simulink model "plant2016_cybership"  (R2015b)
settings: Solver=VariableStepAuto  SolverMode=SingleTasking  StartTime=0.0  StopTime=300  FixedStep=.01  RelTol=1e-3  AbsTol=1e-6
StartFcn:
  | %plot_Contr_index('open')
libraries: simulink x7
(part 1 of 2)
CloseFcn:
  | ;slview('closediagram',bdroot);
settings Model: ExtModeTrigMode=oneshot  ExtModeArmWhenConnect=off  Creator=mjun  LastModifiedBy=TordFO
settings DataIOCC: LimitDataPoints=off  SaveFormat=Array  SignalLoggingSaveFormat=ModelDataLogs  SaveOutput=off  SaveTime=off
settings OptimizationCC: BlockReduction=off  BooleanDataType=off
settings DebuggingCC: SaveWithParameterizedLinksMsg=none  UnderspecifiedInitializationDetection=Classic  MergeDetectMultiDrivingBlocksExec=none  SignalResolutionControl=TryResolveAllWithWarning  MultiTaskDSMMsg=warning  MultiTaskCondExecSysMsg=none
settings HardwareCC: ProdBitPerPointer=32  ProdLargestAtomicFloat=None  ProdIntDivRoundTo=Undefined  ProdEndianess=Unspecified  ProdWordSize=32  ProdHWDeviceType=32-bit Generic  TargetUnknown=on
settings RTWCC: TemplateMakefile=grt_unix.tmf
settings GRTTargetCC: GeneratePreprocessorConditionals=Disable all  CombineOutputUpdateFcns=off  GRTInterface=on
settings ConfigComp: CovModelRefEnable=Off  CovSFcnEnable=off

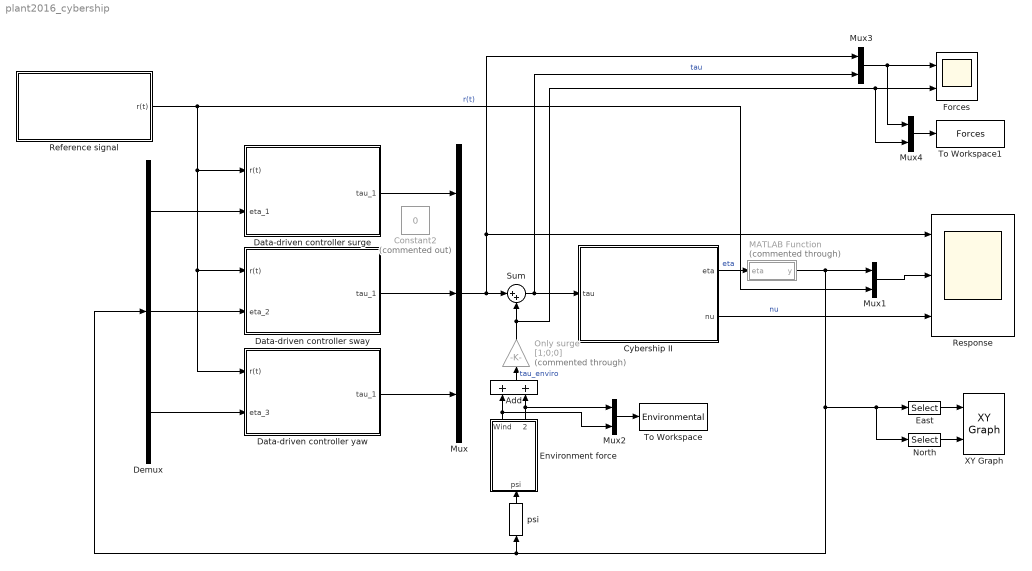
== system plant2016_cybership ==
  Add : Sum
  Constant2 : Constant  Commented=on  Value=0
  Cybership II : Subsystem
  Data-driven controller surge : Subsystem
  Data-driven controller sway : Subsystem
  Data-driven controller yaw : Subsystem
  Demux : Demux  Outputs=3
  East : Selector  InputPortWidth=3  IndexOptions=Index vector (dialog)  Indices=[2]  OutputSizes=1
  Environment force : Subsystem
  Forces : Scope  NumInputPorts=2
  MATLAB Function : MATLAB Function  Commented=through  TreatAsAtomicUnit=on
  Mux : Mux  Inputs=3
  Mux{1..4} (4 alike) : Mux  Inputs=2
  North : Selector  InputPortWidth=3  IndexOptions=Index vector (dialog)  Indices=[1]  OutputSizes=1
  Only surge : Gain  Commented=through  Gain=[1;0;0]
  Reference signal : Subsystem
  Response : Scope  NumInputPorts=3
  Sum : Sum  Inputs=|++
  To Workspace : ToWorkspace  VariableName=Environmental  SaveFormat=Timeseries  SampleTime=-1
  To Workspace1 : ToWorkspace  VariableName=Forces  SaveFormat=Timeseries  SampleTime=-1
  XY Graph : simulink/Sinks/XY Graph  xmin=-1  xmax=1  ymin=-1  ymax=1  st=-1
  psi : Selector  InputPortWidth=3  IndexOptions=Index vector (dialog)  Indices=3  OutputSizes=1
  wires:
  Reference signal/1(r(t)) -> Mux1/2, Data-driven controller sway/1(r(t)), Data-driven controller yaw/1(r(t)), Data-driven controller surge/1(r(t))  "r(t)"
  Mux/1 -> Sum/1, Mux3/1, Response/1
  Cybership II/2(nu) -> Response/3  "nu"
  Demux/3 -> Data-driven controller yaw/2(eta_3)
  Demux/1 -> Data-driven controller surge/2(eta_1)
  Mux1/1 -> Response/2
  Sum/1 -> Mux3/2, Cybership II/1(tau)  "tau"
  Environment force/1(Wind) -> Mux2/2, Add/1
  Environment force/2(Waves) -> Add/2, Mux2/1
  North/1 -> XY Graph/2
  East/1 -> XY Graph/1
  Mux2/1 -> To Workspace/1
  Mux3/1 -> Mux4/1, Forces/1
  Mux4/1 -> To Workspace1/1
  Add/1 -> Only surge/1  "tau_enviro"
  Demux/2 -> Data-driven controller sway/2(eta_2)
  Cybership II/1(eta) -> MATLAB Function/1(eta)  "eta"
  Only surge/1 -> Mux4/2, Forces/2, Sum/2
  Data-driven controller surge/1(tau_1) -> Mux/1
  MATLAB Function/1(y) -> Mux1/1, psi/1, Demux/1, North/1, East/1
  psi/1 -> Environment force/1(psi)
  Data-driven controller yaw/1(tau_1) -> Mux/3
  Data-driven controller sway/1(tau_1) -> Mux/2

== system plant2016_cybership/Cybership II ==
  tau : Inport
  Integrator : Integrator  InitialCondition=[0 0 0]'
  Integrator1 : Integrator  InitialCondition=[0.1;0;0]
  MATLAB Function : MATLAB Function  TreatAsAtomicUnit=on
  Memory : Memory
  Path calculator : MATLAB Function  TreatAsAtomicUnit=on
  Selector : Selector  InputPortWidth=3  IndexOptions=Index vector (dialog)  Indices=3  OutputSizes=1
  To Workspace1 : ToWorkspace  VariableName=nu_dot  SaveFormat=Timeseries  SampleTime=-1
  eta_dot : MATLAB Function  TreatAsAtomicUnit=on
  eta : Outport
  nu : Outport  Port=2
  wires:
  tau/1 -> Path calculator/1(tau)
  eta_dot/1(eta_dot) -> MATLAB Function/1(eta)  "eta_dot"
  Path calculator/1(nu_dot) -> To Workspace1/1, Integrator/1  "nu_dot"
  Integrator1/1 -> Selector/1, eta/1  "eta"
  Integrator/1 -> nu/1, Path calculator/2(nu), eta_dot/2(nu)  "nu"
  Selector/1 -> Memory/1  "psi"
  Memory/1 -> eta_dot/1(psi)  "psi"
  MATLAB Function/1(y) -> Integrator1/1

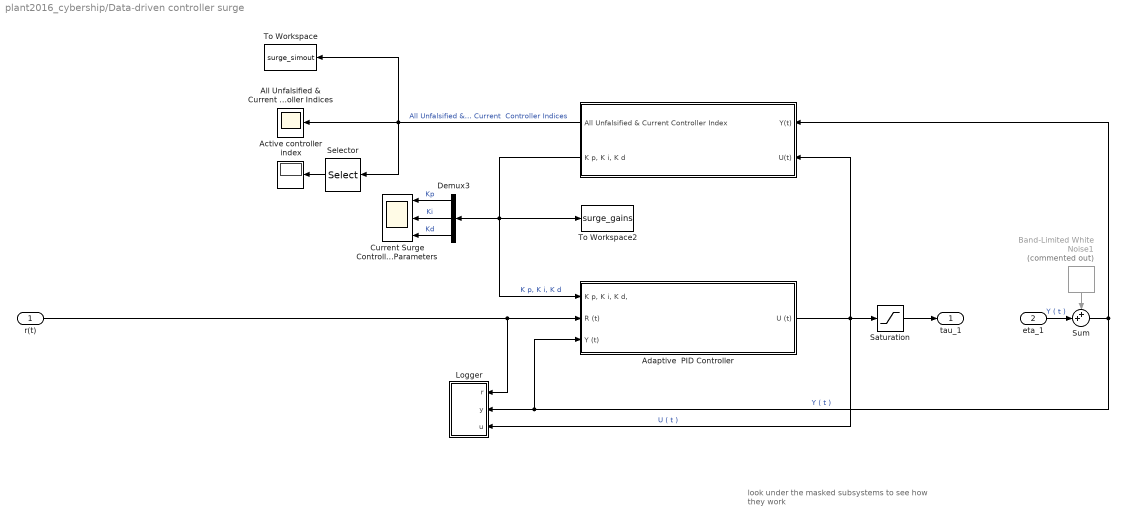
== system plant2016_cybership/Data-driven controller surge ==
  note: look under the masked subsystems
      |  to see how they work
  r(t) : Inport
  eta_1 : Inport  Port=2
  " " : Subsystem  Priority=1  mask(Unfalsification Algorithm){w1_n=1.*[1 20], w1_d=2*[1 3], w2_n=0.01, w2_d=1.2*[1 3 3 1], C_p=[10 100], C_i=[1  20], C_d=[15 20], rho=0.1}
      mask prompts: w1_n "Numerater of filter W1"; w1_d "Denominater of filter W1"; w2_n "Numerater of filter W2"; w2_d "Denominater of filter W2"; C_p "Set of proportional gains, (horizontal vector)"; C_i "Set of integral gains, (horizontal vector)"; C_d "Set of derivative gains, (horizontal vector)"; rho "Set cost-limit"
      mask help:
      | Look under the mask see how "Unfalsification Algorithm" works.
      |
      | Initially, from U & Y, the S-function "fic_ref" generates online the ficticious reference signal for all Candidate Controllers. The S-function "cost_func" then calculates the cost/ performance index for each candidate controllers. Then, based on these Performance Indices, the unfalsification algorithm selects the optimal controller for every instant and outputs the controller parameter ( in our case which is the value of Kp, Ki, Kd).
      |
      | The initilization command of this block calls a m-file "initilization". This m-file sets the port size of the mux & demux blocks inside the subsystem to the number of initial candidate controller whenever the user changes the set of initial condidate controller from the parameter entry block of this subsystem.
      |
      | Original filter-parameters:
      | w1_num =   [1 20]
      | w1_dem = 2*[1 3]
      | w2_num = 0.01
      | w2_den = 1.2*[1 3 3 1]
      mask init:
      | surge_initialization
      mask Help:
      | Look under the mask see how "Unfalsification Algorithm" works.
      | Initially, from U & Y, the S-function "fic_ref" generates online the ficticious reference signal for all Candidate Controllers.
      | The S-function "cost_func" then calculates the cost/ performance index for each candidate controllers.
      | Then, based on these Performance Indices, the S-Function "Supervisor.m" selects the optimal controller for every instant and outputs the controller parameter ( in our case which is the value of Kp, Ki, Kd).
      | The initilization command of this block calls a m-file "initilization". This m-file sets the port size of the mux & demux blocks inside the subsystem to the number of initial candidate controller whenever the user changes the set of initial condidate controller from the parameter entry block of this subsystem.
      mask Display: disp('Unfalsification Algorithm')
  Active controller index : Display
  Adaptive  PID Controller : Subsystem  mask(Adaptive PID Controller){Epsilon=.01, Delta=.010}
      mask prompts: Delta "Sampling time"
      mask init:
      | global epsilon delta
      | epsilon=Epsilon; delta = Delta;
      mask Help: This is an Adaptive PID Controller subsystem. The PID controller parameter (Kp, Ki, Kd) is determined at each instant by the Unfalsification algorithm. Look under the mask to see how this block works. The initilization commands of this block declares "epsilon" & "delta" as global variables. "epsilon" is the time-constant for approximate derivative and "delta" is the sampling time for all s-functions. Other S-functions under the Unfalsification Subsystem access these 2 variables by declaring them as global in their respective m-files.
      mask Display: disp('Adaptive PID Controller')
  All Unfalsified & Current Controller Indices : Scope
      settings: Tag=cont_plot
  Band-Limited White Noise1 : simulink/Sources/Band-Limited White Noise  Commented=on  Cov=[0.00001]  Ts=0.01  seed=[23341]
  Current Surge Controller Parameters : Scope  NumInputPorts=3
  Demux3 : Demux  Outputs=3
  Logger : Subsystem
  Saturation : Saturate  UpperLimit=10  LowerLimit=-10
  Selector : Selector  IndexOptions=Index vector (dialog)  Indices=[1]  OutputSizes=1
  Sum : Sum  Inputs=++|
  To Workspace : ToWorkspace  VariableName=surge_simout  SaveFormat=Timeseries  SampleTime=-1
  To Workspace2 : ToWorkspace  VariableName=surge_gains  SaveFormat=Timeseries  SampleTime=-1
  tau_1 : Outport
  wires:
  " "/1(All Unfalsified & Current Controller Index) -> To Workspace/1, All Unfalsified & Current Controller Indices/1, Selector/1  "All Unfalsified & Current  Controller Indices"
  Adaptive  PID Controller/1(U (t)) -> " "/2(U(t)), Logger/3(u), Saturation/1  "U ( t )"
  " "/2("K p, K i, K d") -> Adaptive  PID Controller/1("K p, K i, K d,"), To Workspace2/1, Demux3/1  "K p, K i, K d"
  Sum/1 -> " "/1(Y(t)), Logger/2(y), Adaptive  PID Controller/3(Y (t))  "Y ( t )"
  Demux3/1 -> Current Surge Controller Parameters/1  "Kp"
  r(t)/1 -> Adaptive  PID Controller/2(R (t)), Logger/1(r)
  eta_1/1 -> Sum/2  "Y ( t )"
  Demux3/2 -> Current Surge Controller Parameters/2  "Ki"
  Band-Limited White Noise1/1 -> Sum/1
  Demux3/3 -> Current Surge Controller Parameters/3  "Kd"
  Selector/1 -> Active controller index/1
  Saturation/1 -> tau_1/1

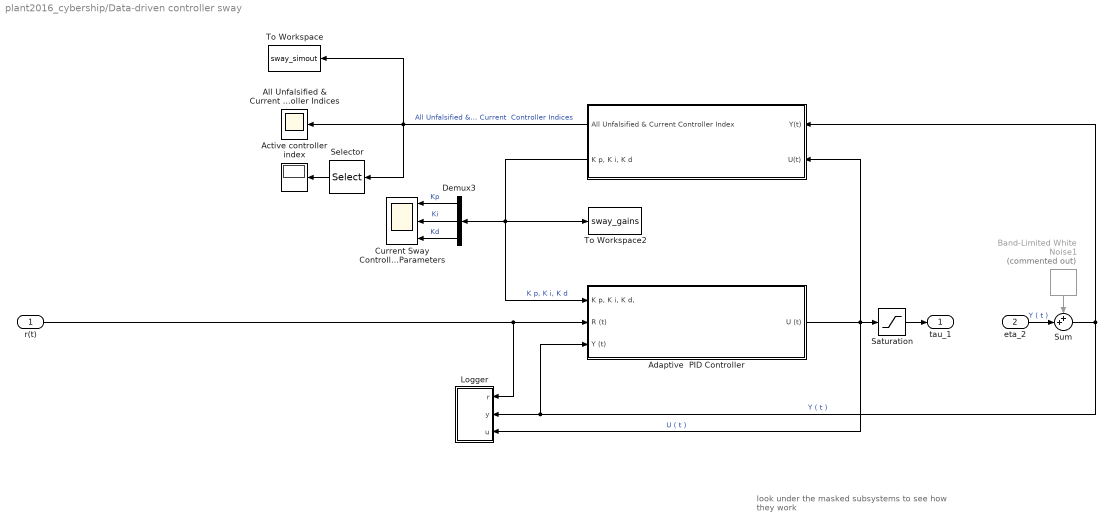
== system plant2016_cybership/Data-driven controller sway ==
  note: look under the masked subsystems
      |  to see how they work
  r(t) : Inport
  eta_2 : Inport  Port=2
  " " : Subsystem  Priority=1  mask(Unfalsification Algorithm){w1_n=1.*[1 20], w1_d=2*[1 3], w2_n=0.01, w2_d=1.2*[1 3 3 1], C_p=[10 150], C_i=[5 10], C_d=[5 10], rho=0.5}
      mask prompts: w1_n "Numerater of filter W1"; w1_d "Denominater of filter W1"; w2_n "Numerater of filter W2"; w2_d "Denominater of filter W2"; C_p "Set of proportional gains, (horizontal vector)"; C_i "Set of integral gains, (horizontal vector)"; C_d "Set of derivative gains, (horizontal vector)"; rho "Set cost-limit"
      mask help:
      | Look under the mask see how "Unfalsification Algorithm" works.
      |
      | Initially, from U & Y, the S-function "fic_ref" generates online the ficticious reference signal for all Candidate Controllers. The S-function "cost_func" then calculates the cost/ performance index for each candidate controllers. Then, based on these Performance Indices, the unfalsification algorithm selects the optimal controller for every instant and outputs the controller parameter ( in our case which is the value of Kp, Ki, Kd).
      |
      | The initilization command of this block calls a m-file "initilization". This m-file sets the port size of the mux & demux blocks inside the subsystem to the number of initial candidate controller whenever the user changes the set of initial condidate controller from the parameter entry block of this subsystem.
      |
      | Original filter-parameters:
      | w1_num =   [1 20]
      | w1_dem = 2*[1 3]
      | w2_num = 0.01
      | w2_den = 1.2*[1 3 3 1]
      mask init:
      | sway_initialization
      mask Help:
      | Look under the mask see how "Unfalsification Algorithm" works.
      | Initially, from U & Y, the S-function "fic_ref" generates online the ficticious reference signal for all Candidate Controllers.
      | The S-function "cost_func" then calculates the cost/ performance index for each candidate controllers.
      | Then, based on these Performance Indices, the S-Function "Supervisor.m" selects the optimal controller for every instant and outputs the controller parameter ( in our case which is the value of Kp, Ki, Kd).
      | The initilization command of this block calls a m-file "initilization". This m-file sets the port size of the mux & demux blocks inside the subsystem to the number of initial candidate controller whenever the user changes the set of initial condidate controller from the parameter entry block of this subsystem.
      mask Display: disp('Unfalsification Algorithm')
  Active controller index : Display
  Adaptive  PID Controller : Subsystem  mask(Adaptive PID Controller){Epsilon=.01, Delta=.01}
      mask prompts: Delta "Sampling time"
      mask init:
      | global epsilon delta
      | epsilon=Epsilon; delta = Delta;
      mask Help: This is an Adaptive PID Controller subsystem. The PID controller parameter (Kp, Ki, Kd) is determined at each instant by the Unfalsification algorithm. Look under the mask to see how this block works. The initilization commands of this block declares "epsilon" & "delta" as global variables. "epsilon" is the time-constant for approximate derivative and "delta" is the sampling time for all s-functions. Other S-functions under the Unfalsification Subsystem access these 2 variables by declaring them as global in their respective m-files.
      mask Display: disp('Adaptive PID Controller')
  All Unfalsified & Current Controller Indices : Scope
      settings: Tag=cont_plot
  Band-Limited White Noise1 : simulink/Sources/Band-Limited White Noise  Commented=on  Cov=[0.00001]  Ts=0.01  seed=[23341]
  Current Sway Controller Parameters : Scope  NumInputPorts=3
  Demux3 : Demux  Outputs=3
  Logger : Subsystem
  Saturation : Saturate  UpperLimit=10  LowerLimit=-10
  Selector : Selector  IndexOptions=Index vector (dialog)  Indices=[1]  OutputSizes=1
  Sum : Sum  Inputs=++|
  To Workspace : ToWorkspace  VariableName=sway_simout  SaveFormat=Timeseries  SampleTime=-1
  To Workspace2 : ToWorkspace  VariableName=sway_gains  SaveFormat=Timeseries  SampleTime=-1
  tau_1 : Outport
  wires:
  Selector/1 -> Active controller index/1
  Demux3/3 -> Current Sway Controller Parameters/3  "Kd"
  Band-Limited White Noise1/1 -> Sum/1
  Demux3/2 -> Current Sway Controller Parameters/2  "Ki"
  eta_2/1 -> Sum/2  "Y ( t )"
  r(t)/1 -> Logger/1(r), Adaptive  PID Controller/2(R (t))
  Demux3/1 -> Current Sway Controller Parameters/1  "Kp"
  Sum/1 -> " "/1(Y(t)), Adaptive  PID Controller/3(Y (t)), Logger/2(y)  "Y ( t )"
  " "/2("K p, K i, K d") -> Demux3/1, To Workspace2/1, Adaptive  PID Controller/1("K p, K i, K d,")  "K p, K i, K d"
  Adaptive  PID Controller/1(U (t)) -> " "/2(U(t)), Saturation/1, Logger/3(u)  "U ( t )"
  " "/1(All Unfalsified & Current Controller Index) -> Selector/1, All Unfalsified & Current Controller Indices/1, To Workspace/1  "All Unfalsified & Current  Controller Indices"
  Saturation/1 -> tau_1/1

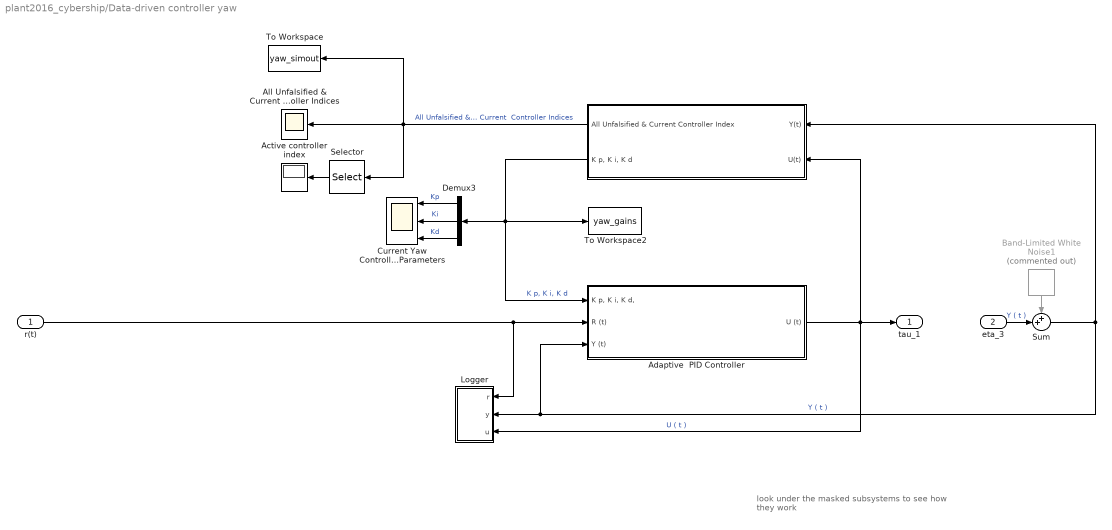
== system plant2016_cybership/Data-driven controller yaw ==
  note: look under the masked subsystems
      |  to see how they work
  r(t) : Inport
  eta_3 : Inport  Port=2
  " " : Subsystem  Priority=1  mask(Unfalsification Algorithm){w1_n=1.*[1 20], w1_d=2*[1 3], w2_n=0.01, w2_d=1.2*[1 3 3 1], C_p=[5 10 20 ], C_i=[1 8], C_d=[5 10], rho=0.2}
      mask prompts: w1_n "Numerater of filter W1"; w1_d "Denominater of filter W1"; w2_n "Numerater of filter W2"; w2_d "Denominater of filter W2"; C_p "Set of proportional gains, (horizontal vector)"; C_i "Set of integral gains, (horizontal vector)"; C_d "Set of derivative gains, (horizontal vector)"; rho "Set cost-limit"
      mask help:
      | Look under the mask see how "Unfalsification Algorithm" works.
      |
      | Initially, from U & Y, the S-function "fic_ref" generates online the ficticious reference signal for all Candidate Controllers. The S-function "cost_func" then calculates the cost/ performance index for each candidate controllers. Then, based on these Performance Indices, the unfalsification algorithm selects the optimal controller for every instant and outputs the controller parameter ( in our case which is the value of Kp, Ki, Kd).
      |
      | The initilization command of this block calls a m-file "initilization". This m-file sets the port size of the mux & demux blocks inside the subsystem to the number of initial candidate controller whenever the user changes the set of initial condidate controller from the parameter entry block of this subsystem.
      |
      | Original filter-parameters:
      | w1_num =   [1 20]
      | w1_dem = 2*[1 3]
      | w2_num = 0.01
      | w2_den = 1.2*[1 3 3 1]
      mask init:
      | yaw_initialization
      mask Help:
      | Look under the mask see how "Unfalsification Algorithm" works.
      | Initially, from U & Y, the S-function "fic_ref" generates online the ficticious reference signal for all Candidate Controllers.
      | The S-function "cost_func" then calculates the cost/ performance index for each candidate controllers.
      | Then, based on these Performance Indices, the S-Function "Supervisor.m" selects the optimal controller for every instant and outputs the controller parameter ( in our case which is the value of Kp, Ki, Kd).
      | The initilization command of this block calls a m-file "initilization". This m-file sets the port size of the mux & demux blocks inside the subsystem to the number of initial candidate controller whenever the user changes the set of initial condidate controller from the parameter entry block of this subsystem.
      mask Display: disp('Unfalsification Algorithm')
  Active controller index : Display
  Adaptive  PID Controller : Subsystem  mask(Adaptive PID Controller){Epsilon=.01, Delta=.01}
      mask prompts: Delta "Sampling time"
      mask init:
      | global epsilon delta
      | epsilon=Epsilon; delta = Delta;
      mask Help: This is an Adaptive PID Controller subsystem. The PID controller parameter (Kp, Ki, Kd) is determined at each instant by the Unfalsification algorithm. Look under the mask to see how this block works. The initilization commands of this block declares "epsilon" & "delta" as global variables. "epsilon" is the time-constant for approximate derivative and "delta" is the sampling time for all s-functions. Other S-functions under the Unfalsification Subsystem access these 2 variables by declaring them as global in their respective m-files.
      mask Display: disp('Adaptive PID Controller')
  All Unfalsified & Current Controller Indices : Scope
      settings: Tag=cont_plot
  Band-Limited White Noise1 : simulink/Sources/Band-Limited White Noise  Commented=on  Cov=[0.00001]  Ts=0.01  seed=[23341]
  Current Yaw Controller Parameters : Scope  NumInputPorts=3
  Demux3 : Demux  Outputs=3
  Logger : Subsystem
  Selector : Selector  IndexOptions=Index vector (dialog)  Indices=[1]  OutputSizes=1
  Sum : Sum  Inputs=++|
  To Workspace : ToWorkspace  VariableName=yaw_simout  SaveFormat=Timeseries  SampleTime=-1
  To Workspace2 : ToWorkspace  VariableName=yaw_gains  SaveFormat=Timeseries  SampleTime=-1
  tau_1 : Outport
  wires:
  " "/1(All Unfalsified & Current Controller Index) -> To Workspace/1, All Unfalsified & Current Controller Indices/1, Selector/1  "All Unfalsified & Current  Controller Indices"
  Adaptive  PID Controller/1(U (t)) -> Logger/3(u), tau_1/1, " "/2(U(t))  "U ( t )"
  " "/2("K p, K i, K d") -> Adaptive  PID Controller/1("K p, K i, K d,"), To Workspace2/1, Demux3/1  "K p, K i, K d"
  Sum/1 -> Logger/2(y), Adaptive  PID Controller/3(Y (t)), " "/1(Y(t))  "Y ( t )"
  Demux3/1 -> Current Yaw Controller Parameters/1  "Kp"
  r(t)/1 -> Adaptive  PID Controller/2(R (t)), Logger/1(r)
  eta_3/1 -> Sum/2  "Y ( t )"
  Demux3/2 -> Current Yaw Controller Parameters/2  "Ki"
  Band-Limited White Noise1/1 -> Sum/1
  Demux3/3 -> Current Yaw Controller Parameters/3  "Kd"
  Selector/1 -> Active controller index/1

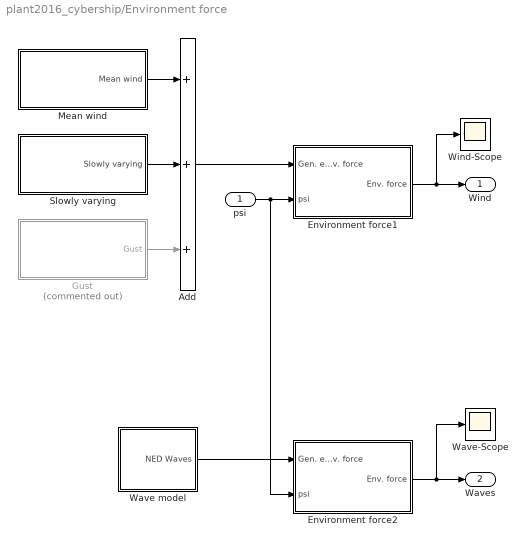
== system plant2016_cybership/Environment force ==
  psi : Inport
  Add : Sum  Inputs=3
  Environment force1 : Subsystem
  Environment force2 : Subsystem
  Gust : Subsystem  Commented=on
  Mean wind : Subsystem  mask{windStrength=5, start=50}
      mask prompts: windStrength "Wind Strength"; start "Start Time"
  Slowly varying : Subsystem  mask{start=70}
      mask prompts: start "Start Time"
  Wave model : Subsystem  mask{start=0, zeta_03=1, omega_01=0.1, omega_02=0.2, omega_03=0.01, zeta_01=0.5, zeta_02=0.5}
      mask prompts: start "Start Time"; zeta_03 "Yaw Damping Ratio"; omega_01 "Dominating Surge Frequency"; omega_02 "Dominating Sway Frequency"; omega_03 "Dominating Yaw Frequency"; zeta_01 "Surge Damping Ratio"; zeta_02 "Sway Damping Ratio"
  Wave-Scope : Scope
  Wind-Scope : Scope
  Wind : Outport
  Waves : Outport  Port=2
  wires:
  Environment force2/1(Env. force) -> Wave-Scope/1, Waves/1
  Add/1 -> Environment force1/1(Gen. env. force)
  Mean wind/1(Mean wind) -> Add/1
  Slowly varying/1(Slowly varying) -> Add/2
  Gust/1(Gust) -> Add/3
  Environment force1/1(Env. force) -> Wind-Scope/1, Wind/1
  psi/1 -> Environment force2/2(psi), Environment force1/2(psi)
  Wave model/1(NED Waves) -> Environment force2/1(Gen. env. force)

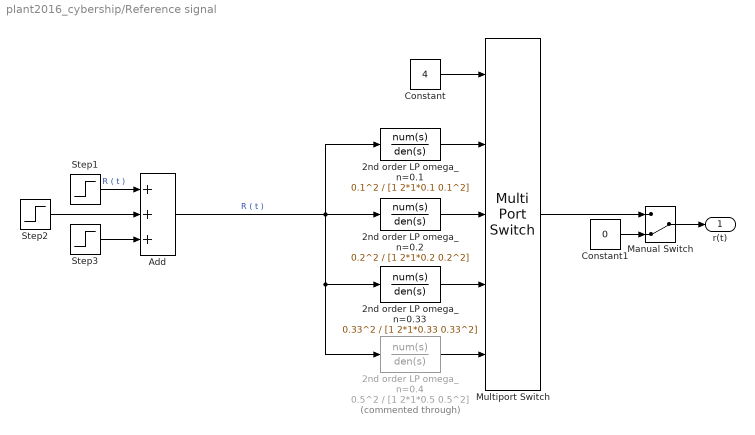
== system plant2016_cybership/Reference signal ==
  2nd order LP omega_n=0.1 : TransferFcn  Numerator=0.1^2  Denominator=[1 2*1*0.1 0.1^2]
  2nd order LP omega_n=0.2 : TransferFcn  Numerator=0.2^2  Denominator=[1 2*1*0.2 0.2^2]
  2nd order LP omega_n=0.33 : TransferFcn  Numerator=0.33^2  Denominator=[1 2*1*0.33 0.33^2]
  2nd order LP omega_n=0.4 : TransferFcn  Commented=through  Numerator=0.5^2  Denominator=[1 2*1*0.5 0.5^2]
  Add : Sum  Inputs=+++
  Constant : Constant  Value=4
  Constant1 : Constant  Value=0
  Manual Switch : ManualSwitch  CurrentSetting=0
  Multiport Switch : MultiPortSwitch  Inputs=4
  Step1 : Step  Time=5  SampleTime=0
  Step2 : Step  Time=30  SampleTime=0
  Step3 : Step  Time=60  After=-2  SampleTime=0
  r(t) : Outport
  wires:
  Add/1 -> 2nd order LP omega_n=0.1/1, 2nd order LP omega_n=0.2/1, 2nd order LP omega_n=0.33/1, 2nd order LP omega_n=0.4/1  "R ( t )"
  Multiport Switch/1 -> Manual Switch/1
  2nd order LP omega_n=0.1/1 -> Multiport Switch/2
  2nd order LP omega_n=0.2/1 -> Multiport Switch/3
  2nd order LP omega_n=0.33/1 -> Multiport Switch/4
  Step1/1 -> Add/1  "R ( t )"
  Step2/1 -> Add/2
  Step3/1 -> Add/3
  2nd order LP omega_n=0.4/1 -> Multiport Switch/5
  Constant/1 -> Multiport Switch/1
  Manual Switch/1 -> r(t)/1
  Constant1/1 -> Manual Switch/2

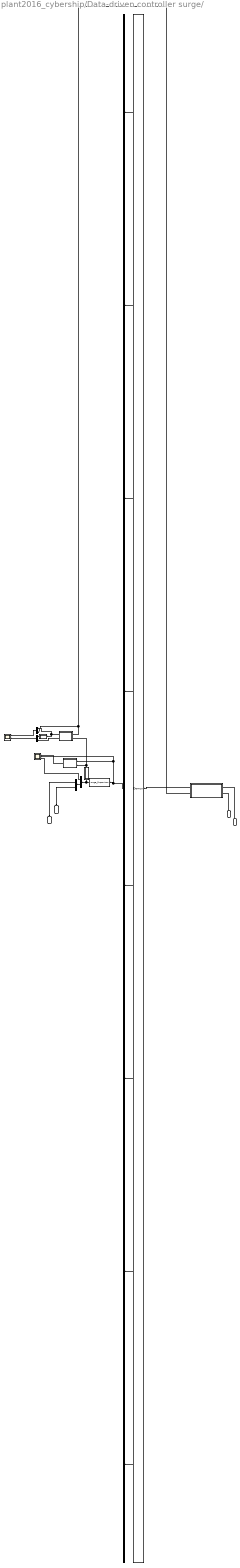
== system plant2016_cybership/Data-driven controller surge/  ==
  note: Performance
      | Index of each
      | Candidate Controller
      | J (n)
  note: n - Candidate Controller Index
  Y(t) : Inport
  U(t) : Inport  Port=2
  Controller Selector : S-Function  FunctionName=surge_Supervisor  Parameters=C_p, C_i, C_d, rho  SFunctionDeploymentMode=off  EnableBusSupport=off
  Cost Surge : Scope  NumInputPorts=3
  Demux. : Demux  Outputs=[3 -1]
  Demux.1 : Demux  Outputs=[1 -1]
  Demux1 : Demux  Tag=surge_demux_1  Outputs=8
  FRS Surge : Scope  NumInputPorts=2
  MATLAB Function : MATLAB Function  TreatAsAtomicUnit=on
  MATLAB Function1 : MATLAB Function  TreatAsAtomicUnit=on
  MATLAB Function2 : MATLAB Function  TreatAsAtomicUnit=on
  Mux : Mux  Inputs=2
  Mux1 : Mux  Tag=surge_mux_1  Inputs=8
  Mux2 : Mux  Inputs=2
  Selector : MATLAB Function  TreatAsAtomicUnit=on
  look under the subsystem to see how it works : Subsystem  Tag=surge_per_monitor
      mask Display: disp('Performance Monitor')
  All Unfalsified & Current Controller Index : Outport  InitialOutput=0
  "K p, K i, K d" : Outport  Port=2  InitialOutput=0
  wires:
  Controller Selector/1 -> Selector/1(u), Demux.1/1
  Demux./1 -> "K p, K i, K d"/1  "Current Controller Parameters"
  Demux./2 -> All Unfalsified & Current Controller Index/1
  Mux1/1 -> Cost Surge/2, MATLAB Function/1(cost), Controller Selector/1  "(n x 1)"
  look under the subsystem to see how it works/1(Out1) -> Demux1/1  "Performance Index of each candidate controller (n x 1)"
  Y(t)/1 -> look under the subsystem to see how it works/1(Y (t))
  U(t)/1 -> look under the subsystem to see how it works/2(U (t))
  Demux.1/2 -> Demux./1
  Demux.1/1 -> Cost Surge/3  "rho"
  Selector/1(y) -> MATLAB Function1/2(i), MATLAB Function/2(i)
  MATLAB Function/1(y) -> Cost Surge/1
  look under the subsystem to see how it works/2(frs) -> MATLAB Function1/1(frs), Mux/2
  MATLAB Function1/1(y) -> MATLAB Function2/1(u), Mux/1
  MATLAB Function1/2(y_sqr) -> Mux2/2
  Mux/1 -> FRS Surge/1  "FRS"
  Mux2/1 -> FRS Surge/2  "FRS squared"
  MATLAB Function2/1(y) -> Mux2/1
  Demux1/1 -> Mux1/1
  Demux1/2 -> Mux1/2
  Demux1/3 -> Mux1/3
  Demux1/4 -> Mux1/4
  Demux1/5 -> Mux1/5
  Demux1/6 -> Mux1/6
  Demux1/7 -> Mux1/7
  Demux1/8 -> Mux1/8

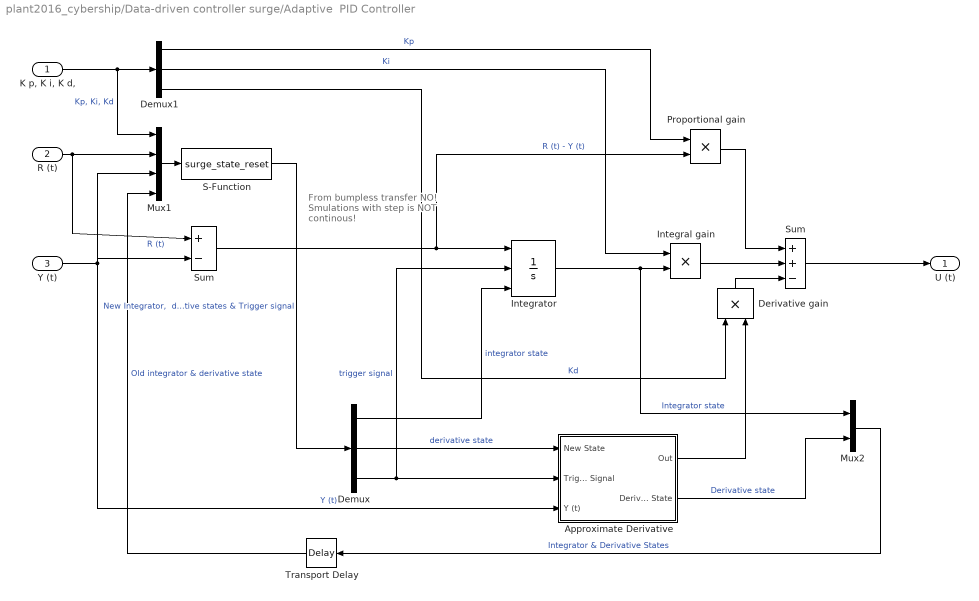
== system plant2016_cybership/Data-driven controller surge/Adaptive  PID Controller ==
  note: From bumpless transfer
      | NO! Smulations
      | with step is NOT
      | continous!
  "K p, K i, K d," : Inport
  R (t) : Inport  Port=2
  Y (t) : Inport  Port=3
  Approximate Derivative : Subsystem
  Demux : Demux  Outputs=3
  Demux1 : Demux  Outputs=3
  Derivative gain : Product  SaturateOnIntegerOverflow=on  RndMeth=Zero  InputSameDT=on  OutDataTypeStr=Inherit: Same as first input
  Integral gain : Product  SaturateOnIntegerOverflow=on  RndMeth=Zero  InputSameDT=on  OutDataTypeStr=Inherit: Same as first input
  Integrator : Integrator  ExternalReset=either  InitialConditionSource=external
  Mux1 : Mux
  Mux2 : Mux  Inputs=2
  Proportional gain : Product  SaturateOnIntegerOverflow=on  RndMeth=Zero  InputSameDT=on  OutDataTypeStr=Inherit: Same as first input
  S-Function : S-Function  FunctionName=surge_state_reset  Parameters=epsilon, delta  SFunctionDeploymentMode=off  EnableBusSupport=off
      mask Help:
      | S function, inside "Adaptive PID Controller" block, for resetting the
      | controller state, when switching to a new controller, in order to reduce unwanted abrupt peaks in control signal u(t). Also generates trigger signal for the same purpose.
  Sum : Sum  Inputs=++-  SaturateOnIntegerOverflow=on  InputSameDT=on  OutDataTypeStr=Inherit: Same as first input
  "Sum " : Sum  Inputs=+|-  SaturateOnIntegerOverflow=on  InputSameDT=on  OutDataTypeStr=Inherit: Same as first input
  Transport Delay : TransportDelay  DelayTime=delta
  U (t) : Outport  InitialOutput=0
  wires:
  Proportional gain/1 -> Sum/1
  Approximate Derivative/1(Out) -> Derivative gain/2
  Integral gain/1 -> Sum/2
  Derivative gain/1 -> Sum/3
  Integrator/1 -> Integral gain/2, Mux2/1  "Integrator state"
  "Sum "/1 -> Integrator/1, Proportional gain/2  "R (t) - Y (t)"
  Sum/1 -> U (t)/1
  Demux1/2 -> Integral gain/1  "Ki"
  Demux1/1 -> Proportional gain/1  "Kp"
  Demux/1 -> Integrator/3  "integrator state"
  Approximate Derivative/2(Derivative State) -> Mux2/2  "Derivative state"
  Demux/2 -> Approximate Derivative/1(New State)  "derivative state"
  Demux1/3 -> Derivative gain/1  "Kd"
  S-Function/1 -> Demux/1  "New Integrator,  derivative states & Trigger signal"
  Mux1/1 -> S-Function/1
  R (t)/1 -> Mux1/2, "Sum "/1  "R (t)"
  "K p, K i, K d,"/1 -> Mux1/1, Demux1/1  "Kp, Ki, Kd"
  Mux2/1 -> Transport Delay/1  "Integrator & Derivative States"
  Transport Delay/1 -> Mux1/4  "Old integrator & derivative state"
  Demux/3 -> Integrator/2, Approximate Derivative/2(Trigger Signal)  "trigger signal"
  Y (t)/1 -> "Sum "/2, Mux1/3, Approximate Derivative/3(Y (t))  "Y (t)"

== system plant2016_cybership/Data-driven controller surge/Logger ==
  r : Inport
  y : Inport  Port=2
  u : Inport  Port=3
  Mux1 : Mux
  Subtract : Sum  Inputs=+-
  To Workspace1 : ToWorkspace  VariableName=surge_result  SaveFormat=Timeseries  SampleTime=-1
  wires:
  Mux1/1 -> To Workspace1/1
  Subtract/1 -> Mux1/3  "e"
  u/1 -> Mux1/4  "u"
  r/1 -> Mux1/1, Subtract/2  "r"
  y/1 -> Mux1/2, Subtract/1  "y"

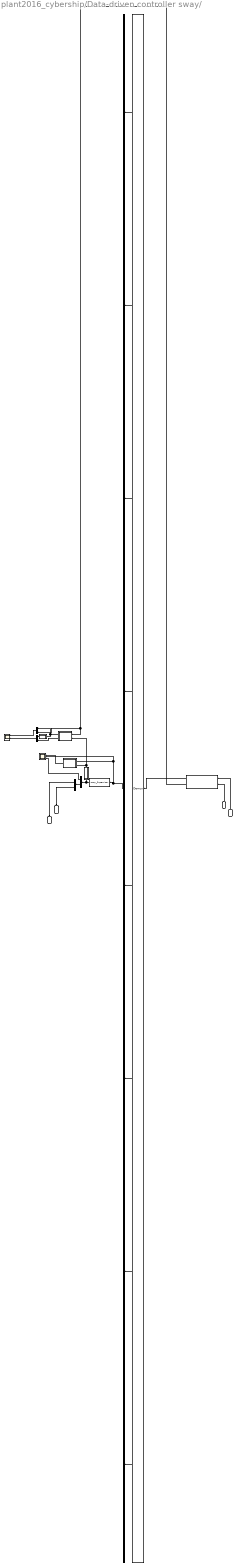
== system plant2016_cybership/Data-driven controller sway/  ==
  note: n - Candidate Controller Index
  note: Performance
      | Index of each
      | Candidate Controller
      | J (n)
  Y(t) : Inport
  U(t) : Inport  Port=2
  Controller Selector : S-Function  FunctionName=sway_Supervisor  Parameters=C_p, C_i, C_d, rho  SFunctionDeploymentMode=off  EnableBusSupport=off
  Cost Sway : Scope  NumInputPorts=3
  Demux. : Demux  Outputs=[3 -1]
  Demux.1 : Demux  Outputs=[1 -1]
  Demux1 : Demux  Tag=sway_demux_1  Outputs=8
  FRS Sway : Scope  NumInputPorts=2
  MATLAB Function : MATLAB Function  TreatAsAtomicUnit=on
  MATLAB Function1 : MATLAB Function  TreatAsAtomicUnit=on
  MATLAB Function2 : MATLAB Function  TreatAsAtomicUnit=on
  Mux : Mux  Inputs=2
  Mux1 : Mux  Tag=sway_mux_1  Inputs=8
  Mux2 : Mux  Inputs=2
  Selector : MATLAB Function  TreatAsAtomicUnit=on
  look under the subsystem to see how it works : Subsystem  Tag=sway_per_monitor
      mask Display: disp('Performance Monitor')
  All Unfalsified & Current Controller Index : Outport  InitialOutput=0
  "K p, K i, K d" : Outport  Port=2  InitialOutput=0
  wires:
  MATLAB Function2/1(y) -> Mux2/1
  Mux2/1 -> FRS Sway/2  "FRS squared"
  Mux/1 -> FRS Sway/1  "FRS"
  MATLAB Function1/2(y_sqr) -> Mux2/2
  MATLAB Function1/1(y) -> MATLAB Function2/1(u), Mux/1
  look under the subsystem to see how it works/2(frs) -> MATLAB Function1/1(frs), Mux/2
  MATLAB Function/1(y) -> Cost Sway/1
  Selector/1(y) -> MATLAB Function/2(i), MATLAB Function1/2(i)
  Demux.1/1 -> Cost Sway/3  "rho"
  Demux.1/2 -> Demux./1
  U(t)/1 -> look under the subsystem to see how it works/2(U (t))
  Y(t)/1 -> look under the subsystem to see how it works/1(Y (t))
  look under the subsystem to see how it works/1(Out1) -> Demux1/1  "Performance Index of each candidate controller (n x 1)"
  Mux1/1 -> Controller Selector/1, Cost Sway/2, MATLAB Function/1(cost)  "(n x 1)"
  Demux./2 -> All Unfalsified & Current Controller Index/1
  Demux./1 -> "K p, K i, K d"/1  "Current Controller Parameters"
  Controller Selector/1 -> Demux.1/1, Selector/1(u)
  Demux1/1 -> Mux1/1
  Demux1/2 -> Mux1/2
  Demux1/3 -> Mux1/3
  Demux1/4 -> Mux1/4
  Demux1/5 -> Mux1/5
  Demux1/6 -> Mux1/6
  Demux1/7 -> Mux1/7
  Demux1/8 -> Mux1/8

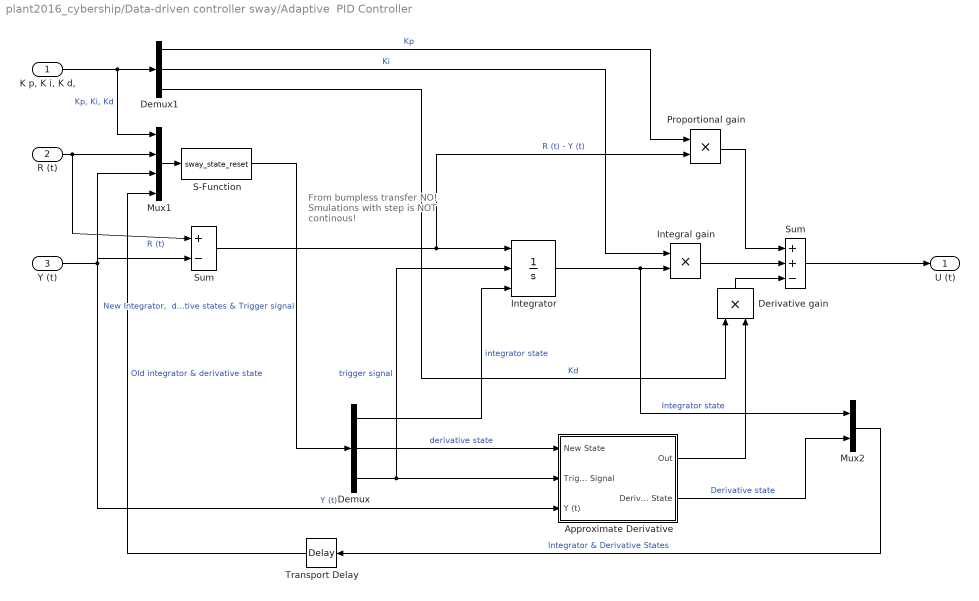
== system plant2016_cybership/Data-driven controller sway/Adaptive  PID Controller ==
  note: From bumpless transfer
      | NO! Smulations
      | with step is NOT
      | continous!
  "K p, K i, K d," : Inport
  R (t) : Inport  Port=2
  Y (t) : Inport  Port=3
  Approximate Derivative : Subsystem
  Demux : Demux  Outputs=3
  Demux1 : Demux  Outputs=3
  Derivative gain : Product  SaturateOnIntegerOverflow=on  RndMeth=Zero  InputSameDT=on  OutDataTypeStr=Inherit: Same as first input
  Integral gain : Product  SaturateOnIntegerOverflow=on  RndMeth=Zero  InputSameDT=on  OutDataTypeStr=Inherit: Same as first input
  Integrator : Integrator  ExternalReset=either  InitialConditionSource=external
  Mux1 : Mux
  Mux2 : Mux  Inputs=2
  Proportional gain : Product  SaturateOnIntegerOverflow=on  RndMeth=Zero  InputSameDT=on  OutDataTypeStr=Inherit: Same as first input
  S-Function : S-Function  FunctionName=sway_state_reset  Parameters=epsilon, delta  SFunctionDeploymentMode=off  EnableBusSupport=off
      mask Help:
      | S function, inside "Adaptive PID Controller" block, for resetting the
      | controller state, when switching to a new controller, in order to reduce unwanted abrupt peaks in control signal u(t). Also generates trigger signal for the same purpose.
  Sum : Sum  Inputs=++-  SaturateOnIntegerOverflow=on  InputSameDT=on  OutDataTypeStr=Inherit: Same as first input
  "Sum " : Sum  Inputs=+|-  SaturateOnIntegerOverflow=on  InputSameDT=on  OutDataTypeStr=Inherit: Same as first input
  Transport Delay : TransportDelay  DelayTime=delta
  U (t) : Outport  InitialOutput=0
  wires:
  Y (t)/1 -> Approximate Derivative/3(Y (t)), Mux1/3, "Sum "/2  "Y (t)"
  Demux/3 -> Approximate Derivative/2(Trigger Signal), Integrator/2  "trigger signal"
  Transport Delay/1 -> Mux1/4  "Old integrator & derivative state"
  Mux2/1 -> Transport Delay/1  "Integrator & Derivative States"
  "K p, K i, K d,"/1 -> Demux1/1, Mux1/1  "Kp, Ki, Kd"
  R (t)/1 -> "Sum "/1, Mux1/2  "R (t)"
  Mux1/1 -> S-Function/1
  S-Function/1 -> Demux/1  "New Integrator,  derivative states & Trigger signal"
  Demux1/3 -> Derivative gain/1  "Kd"
  Demux/2 -> Approximate Derivative/1(New State)  "derivative state"
  Approximate Derivative/2(Derivative State) -> Mux2/2  "Derivative state"
  Demux/1 -> Integrator/3  "integrator state"
  Demux1/1 -> Proportional gain/1  "Kp"
  Demux1/2 -> Integral gain/1  "Ki"
  Sum/1 -> U (t)/1
  "Sum "/1 -> Proportional gain/2, Integrator/1  "R (t) - Y (t)"
  Integrator/1 -> Mux2/1, Integral gain/2  "Integrator state"
  Derivative gain/1 -> Sum/3
  Integral gain/1 -> Sum/2
  Approximate Derivative/1(Out) -> Derivative gain/2
  Proportional gain/1 -> Sum/1

== system plant2016_cybership/Data-driven controller sway/Logger ==
  r : Inport
  y : Inport  Port=2
  u : Inport  Port=3
  Mux1 : Mux
  Subtract : Sum  Inputs=+-
  To Workspace1 : ToWorkspace  VariableName=sway_result  SaveFormat=Timeseries  SampleTime=-1
  wires:
  y/1 -> Subtract/1, Mux1/2  "y"
  r/1 -> Subtract/2, Mux1/1  "r"
  u/1 -> Mux1/4  "u"
  Subtract/1 -> Mux1/3  "e"
  Mux1/1 -> To Workspace1/1

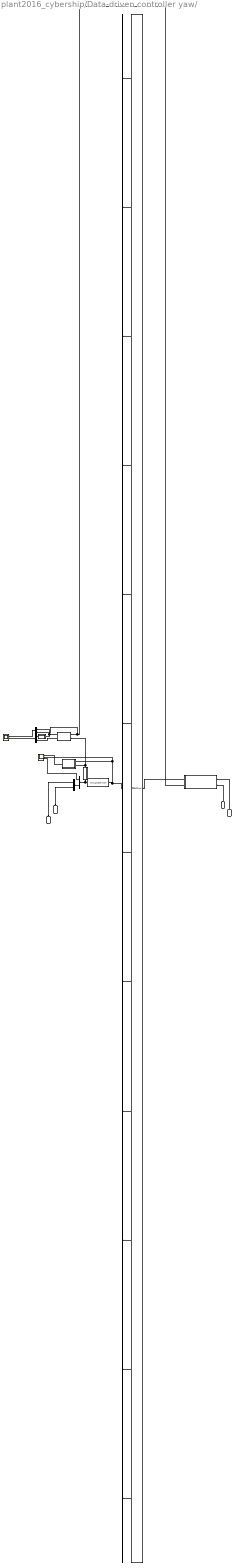
== system plant2016_cybership/Data-driven controller yaw/  ==
  note: Performance
      | Index of each
      | Candidate Controller
      | J (n)
  note: n - Candidate Controller Index
  Y(t) : Inport
  U(t) : Inport  Port=2
  Controller Selector : S-Function  FunctionName=yaw_Supervisor  Parameters=C_p, C_i, C_d, rho  SFunctionDeploymentMode=off  EnableBusSupport=off
  Cost : Scope  NumInputPorts=3
  Demux. : Demux  Outputs=[3 -1]
  Demux.1 : Demux  Outputs=[1 -1]
  Demux1 : Demux  Tag=yaw_demux_1  Outputs=12
  FRS : Scope  NumInputPorts=2
  MATLAB Function : MATLAB Function  TreatAsAtomicUnit=on
  MATLAB Function1 : MATLAB Function  TreatAsAtomicUnit=on
  MATLAB Function2 : MATLAB Function  TreatAsAtomicUnit=on
  Mux : Mux  Inputs=2
  Mux1 : Mux  Tag=yaw_mux_1  Inputs=12
  Mux2 : Mux  Inputs=2
  Selector : MATLAB Function  TreatAsAtomicUnit=on
  look under the subsystem to see how it works : Subsystem  Tag=yaw_per_monitor
      mask Display: disp('Performance Monitor')
  All Unfalsified & Current Controller Index : Outport  InitialOutput=0
  "K p, K i, K d" : Outport  Port=2  InitialOutput=0
  wires:
  Controller Selector/1 -> Selector/1(u), Demux.1/1
  Demux./1 -> "K p, K i, K d"/1  "Current Controller Parameters"
  Demux./2 -> All Unfalsified & Current Controller Index/1
  Mux1/1 -> Cost/2, MATLAB Function/1(cost), Controller Selector/1  "(n x 1)"
  look under the subsystem to see how it works/1(Out1) -> Demux1/1  "Performance Index of each candidate controller (n x 1)"
  Y(t)/1 -> look under the subsystem to see how it works/1(Y (t))
  U(t)/1 -> look under the subsystem to see how it works/2(U (t))
  Demux.1/2 -> Demux./1
  Demux.1/1 -> Cost/3  "rho"
  Selector/1(y) -> MATLAB Function1/2(i), MATLAB Function/2(i)
  MATLAB Function/1(y) -> Cost/1
  look under the subsystem to see how it works/2(frs) -> Mux/2, MATLAB Function1/1(frs)
  MATLAB Function1/1(y) -> MATLAB Function2/1(u), Mux/1
  MATLAB Function1/2(y_sqr) -> Mux2/2
  Mux/1 -> FRS/1  "FRS"
  Mux2/1 -> FRS/2  "FRS squared"
  MATLAB Function2/1(y) -> Mux2/1
  Demux1/1 -> Mux1/1
  Demux1/2 -> Mux1/2
  Demux1/3 -> Mux1/3
  Demux1/4 -> Mux1/4
  Demux1/5 -> Mux1/5
  Demux1/6 -> Mux1/6
  Demux1/7 -> Mux1/7
  Demux1/8 -> Mux1/8
  Demux1/9 -> Mux1/9
  Demux1/10 -> Mux1/10
  Demux1/11 -> Mux1/11
  Demux1/12 -> Mux1/12

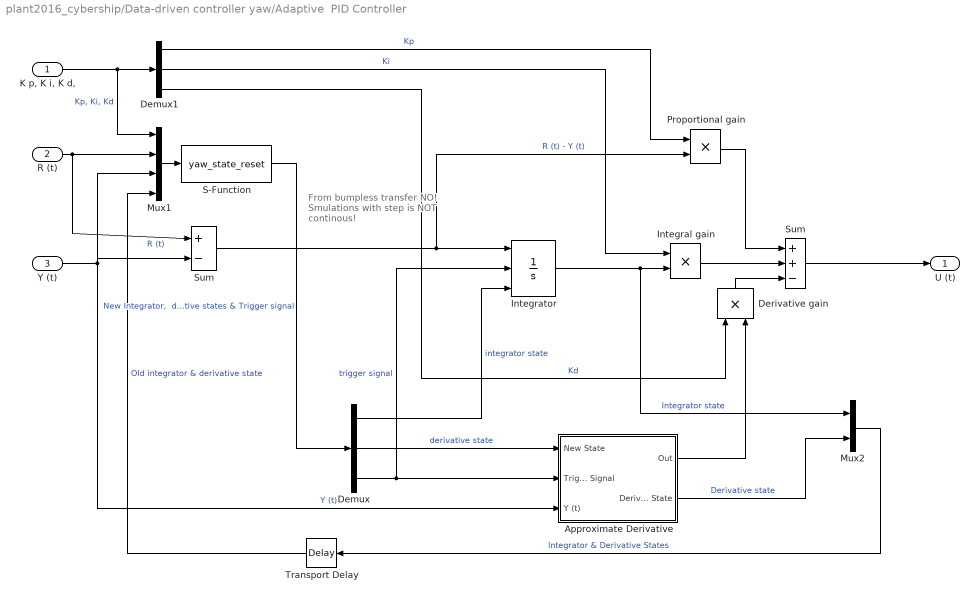
== system plant2016_cybership/Data-driven controller yaw/Adaptive  PID Controller ==
  note: From bumpless transfer
      | NO! Smulations
      | with step is NOT
      | continous!
  "K p, K i, K d," : Inport
  R (t) : Inport  Port=2
  Y (t) : Inport  Port=3
  Approximate Derivative : Subsystem
  Demux : Demux  Outputs=3
  Demux1 : Demux  Outputs=3
  Derivative gain : Product  SaturateOnIntegerOverflow=on  RndMeth=Zero  InputSameDT=on  OutDataTypeStr=Inherit: Same as first input
  Integral gain : Product  SaturateOnIntegerOverflow=on  RndMeth=Zero  InputSameDT=on  OutDataTypeStr=Inherit: Same as first input
  Integrator : Integrator  ExternalReset=either  InitialConditionSource=external
  Mux1 : Mux
  Mux2 : Mux  Inputs=2
  Proportional gain : Product  SaturateOnIntegerOverflow=on  RndMeth=Zero  InputSameDT=on  OutDataTypeStr=Inherit: Same as first input
  S-Function : S-Function  FunctionName=yaw_state_reset  Parameters=epsilon, delta  SFunctionDeploymentMode=off  EnableBusSupport=off
      mask Help:
      | S function, inside "Adaptive PID Controller" block, for resetting the
      | controller state, when switching to a new controller, in order to reduce unwanted abrupt peaks in control signal u(t). Also generates trigger signal for the same purpose.
  Sum : Sum  Inputs=++-  SaturateOnIntegerOverflow=on  InputSameDT=on  OutDataTypeStr=Inherit: Same as first input
  "Sum " : Sum  Inputs=+|-  SaturateOnIntegerOverflow=on  InputSameDT=on  OutDataTypeStr=Inherit: Same as first input
  Transport Delay : TransportDelay  DelayTime=delta
  U (t) : Outport  InitialOutput=0
  wires:
  Proportional gain/1 -> Sum/1
  Approximate Derivative/1(Out) -> Derivative gain/2
  Integral gain/1 -> Sum/2
  Derivative gain/1 -> Sum/3
  Integrator/1 -> Integral gain/2, Mux2/1  "Integrator state"
  "Sum "/1 -> Integrator/1, Proportional gain/2  "R (t) - Y (t)"
  Sum/1 -> U (t)/1
  Demux1/2 -> Integral gain/1  "Ki"
  Demux1/1 -> Proportional gain/1  "Kp"
  Demux/1 -> Integrator/3  "integrator state"
  Approximate Derivative/2(Derivative State) -> Mux2/2  "Derivative state"
  Demux/2 -> Approximate Derivative/1(New State)  "derivative state"
  Demux1/3 -> Derivative gain/1  "Kd"
  S-Function/1 -> Demux/1  "New Integrator,  derivative states & Trigger signal"
  Mux1/1 -> S-Function/1
  R (t)/1 -> Mux1/2, "Sum "/1  "R (t)"
  "K p, K i, K d,"/1 -> Mux1/1, Demux1/1  "Kp, Ki, Kd"
  Mux2/1 -> Transport Delay/1  "Integrator & Derivative States"
  Transport Delay/1 -> Mux1/4  "Old integrator & derivative state"
  Demux/3 -> Integrator/2, Approximate Derivative/2(Trigger Signal)  "trigger signal"
  Y (t)/1 -> "Sum "/2, Mux1/3, Approximate Derivative/3(Y (t))  "Y (t)"

== system plant2016_cybership/Data-driven controller yaw/Logger ==
  r : Inport
  y : Inport  Port=2
  u : Inport  Port=3
  Mux1 : Mux
  Subtract : Sum  Inputs=+-
  To Workspace1 : ToWorkspace  VariableName=yaw_result  SaveFormat=Timeseries  SampleTime=-1
  wires:
  Mux1/1 -> To Workspace1/1
  Subtract/1 -> Mux1/3  "e"
  u/1 -> Mux1/4  "u"
  r/1 -> Mux1/1, Subtract/2  "r"
  y/1 -> Mux1/2, Subtract/1  "y"

== system plant2016_cybership/Environment force/Environment force1 ==
  Gen. env. force : Inport
  psi : Inport  Port=2
  Scope : Scope
  Wind direction : Subsystem
  Wind force : MATLAB Function  TreatAsAtomicUnit=on
  r2d : Gain  Gain=180/pi
  Env. force : Outport
  wires:
  Gen. env. force/1 -> Wind force/3(u)
  Wind force/1(y) -> Env. force/1
  psi/1 -> Wind force/2(psi)
  Wind direction/1(beta_w) -> r2d/1, Wind force/1(beta_w)
  r2d/1 -> Scope/1

== system plant2016_cybership/Environment force/Environment force2 ==
  Gen. env. force : Inport
  psi : Inport  Port=2
  NED2Body : MATLAB Function  TreatAsAtomicUnit=on
  Env. force : Outport
  wires:
  psi/1 -> NED2Body/1(psi)
  NED2Body/1(y) -> Env. force/1
  Gen. env. force/1 -> NED2Body/2(u)

== system plant2016_cybership/Environment force/Gust ==
  Constant : Constant  Value=0
  Gust : Outport
  wires:
  Constant/1 -> Gust/1

== system plant2016_cybership/Environment force/Mean wind ==
  Constant4 : Constant  Value=windStrength
  Product : Product
  Reference filter : Subsystem
  Start1 : Step  Time=start  SampleTime=0
  Mean wind : Outport
  wires:
  Constant4/1 -> Product/2
  Start1/1 -> Product/1
  Reference filter/1(r) -> Mean wind/1  "mean_wind"
  Product/1 -> Reference filter/1(r(t))

== system plant2016_cybership/Environment force/Slowly varying ==
  1st order Markov2 : Subsystem
  Band-Limited White Noise1 : simulink/Sources/Band-Limited White Noise  Cov=1  Ts=0.1  seed=[23341]
  Product : Product
  Scope : Scope
  Start1 : Step  Time=100  SampleTime=0
  Slowly varying : Outport
  wires:
  Product/1 -> Scope/1, Slowly varying/1  "Slowly"
  Start1/1 -> Product/1
  1st order Markov2/1(Out1) -> Product/2
  Band-Limited White Noise1/1 -> 1st order Markov2/1(In1)

== system plant2016_cybership/Environment force/Wave model ==
  2nd order Markov : Subsystem
  Band-Limited White Noise1 : simulink/Sources/Band-Limited White Noise  Cov=[0.1;0.1;0.01]  Ts=0.1  seed=[23341]
  Product : Product
  Step : Step  Time=start  SampleTime=0
  NED Waves : Outport
  wires:
  Band-Limited White Noise1/1 -> 2nd order Markov/1(wn)
  2nd order Markov/1(out) -> Product/2
  Product/1 -> NED Waves/1
  Step/1 -> Product/1

== system plant2016_cybership/Data-driven controller surge/ /look under the subsystem to see how it works ==
  note: Ficticious Reference
      | Signal of individual
      | Candidate Controller
      | R_fict (n)
  note: n - Candidate Controller Index
  Y (t) : Inport
  U (t) : Inport  Port=2
  Cost / Performance Index Generator : S-Function  FunctionName=surge_cost_func  Parameters=w1_n, w1_d, w2_n, w2_d, C_p, C_i, C_d  SFunctionDeploymentMode=off  EnableBusSupport=off
  Demux2 : Demux  Tag=surge_demux_2  Outputs=8
  Ficticious Reference Signal Generator : S-Function  FunctionName=surge_fic_ref  Parameters=C_p, C_i, C_d  SFunctionDeploymentMode=off  EnableBusSupport=off
  Mux. : Mux  Inputs=2
  Mux.. : Mux  Inputs=2
  Mux2 : Mux  Tag=surge_mux_2  Inputs=8
  To Workspace : ToWorkspace  VariableName=surge_frs  SaveFormat=Timeseries  SampleTime=-1
  To Workspace1 : ToWorkspace  VariableName=surge_cost  SaveFormat=Timeseries  SampleTime=-1
  Out1 : Outport
  frs : Outport  Port=2
  wires:
  U (t)/1 -> Mux../1
  Mux./1 -> Cost / Performance Index Generator/1  "(r_fict(t), u(t), y(t))"
  Mux../1 -> Ficticious Reference Signal Generator/1, Mux./1  "U & Y"
  Y (t)/1 -> Mux../2
  Ficticious Reference Signal Generator/1 -> frs/1, To Workspace/1, Demux2/1
  Mux2/1 -> Mux./2  "R_Fict ( n x 1 )"
  Cost / Performance Index Generator/1 -> To Workspace1/1, Out1/1  "Performance Index of  each candidate controller (n x 1)"
  Demux2/1 -> Mux2/1
  Demux2/2 -> Mux2/2
  Demux2/3 -> Mux2/3
  Demux2/4 -> Mux2/4
  Demux2/5 -> Mux2/5
  Demux2/6 -> Mux2/6
  Demux2/7 -> Mux2/7
  Demux2/8 -> Mux2/8

== system plant2016_cybership/Data-driven controller surge/Adaptive  PID Controller/Approximate Derivative ==
  New State : Inport
  Trigger Signal : Inport  Port=2
  Y (t) : Inport  Port=3
  Gain : Gain  Gain=1/epsilon^2  SaturateOnIntegerOverflow=on  OutDataTypeStr=Inherit: Same as input  ParamDataTypeStr=Inherit: Same as input
  Gain1 : Gain  Gain=1/epsilon  SaturateOnIntegerOverflow=on  OutDataTypeStr=Inherit: Same as input  ParamDataTypeStr=Inherit: Same as input
  Gain2 : Gain  Gain=1/epsilon  SaturateOnIntegerOverflow=on  OutDataTypeStr=Inherit: Same as input  ParamDataTypeStr=Inherit: Same as input
  Integrator : Integrator  ExternalReset=either  InitialConditionSource=external
  Sum : Sum  Inputs=+-  SaturateOnIntegerOverflow=on  InputSameDT=on  OutDataTypeStr=Inherit: Same as first input
  Sum1 : Sum  Inputs=+-  SaturateOnIntegerOverflow=on  InputSameDT=on  OutDataTypeStr=Inherit: Same as first input
  Out : Outport
  Derivative State : Outport  Port=2
  wires:
  Sum/1 -> Integrator/1
  Y (t)/1 -> Gain1/1, Sum/1
  Gain1/1 -> Sum1/1
  Gain2/1 -> Sum/2
  Sum1/1 -> Out/1
  New State/1 -> Integrator/3
  Trigger Signal/1 -> Integrator/2
  Gain/1 -> Sum1/2
  Integrator/1 -> Derivative State/1, Gain2/1, Gain/1

== system plant2016_cybership/Data-driven controller sway/ /look under the subsystem to see how it works ==
  note: n - Candidate Controller Index
  note: Ficticious Reference
      | Signal of individual
      | Candidate Controller
      | R_fict (n)
  Y (t) : Inport
  U (t) : Inport  Port=2
  Cost / Performance Index Generator : S-Function  FunctionName=sway_cost_func  Parameters=w1_n, w1_d, w2_n, w2_d, C_p, C_i, C_d  SFunctionDeploymentMode=off  EnableBusSupport=off
  Demux2 : Demux  Tag=sway_demux_2  Outputs=8
  Ficticious Reference Signal Generator : S-Function  FunctionName=sway_fic_ref  Parameters=C_p, C_i, C_d  SFunctionDeploymentMode=off  EnableBusSupport=off
  Mux. : Mux  Inputs=2
  Mux.. : Mux  Inputs=2
  Mux2 : Mux  Tag=sway_mux_2  Inputs=8
  To Workspace : ToWorkspace  VariableName=sway_frs  SaveFormat=Timeseries  SampleTime=-1
  To Workspace1 : ToWorkspace  VariableName=sway_cost  SaveFormat=Timeseries  SampleTime=-1
  Out1 : Outport
  frs : Outport  Port=2
  wires:
  Cost / Performance Index Generator/1 -> Out1/1, To Workspace1/1  "Performance Index of  each candidate controller (n x 1)"
  Mux2/1 -> Mux./2  "R_Fict ( n x 1 )"
  Ficticious Reference Signal Generator/1 -> Demux2/1, To Workspace/1, frs/1
  Y (t)/1 -> Mux../2
  Mux../1 -> Mux./1, Ficticious Reference Signal Generator/1  "U & Y"
  Mux./1 -> Cost / Performance Index Generator/1  "(r_fict(t), u(t), y(t))"
  U (t)/1 -> Mux../1
  Demux2/1 -> Mux2/1
  Demux2/2 -> Mux2/2
  Demux2/3 -> Mux2/3
  Demux2/4 -> Mux2/4
  Demux2/5 -> Mux2/5
  Demux2/6 -> Mux2/6
  Demux2/7 -> Mux2/7
  Demux2/8 -> Mux2/8

== system plant2016_cybership/Data-driven controller sway/Adaptive  PID Controller/Approximate Derivative ==
  New State : Inport
  Trigger Signal : Inport  Port=2
  Y (t) : Inport  Port=3
  Gain : Gain  Gain=1/epsilon^2  SaturateOnIntegerOverflow=on  OutDataTypeStr=Inherit: Same as input  ParamDataTypeStr=Inherit: Same as input
  Gain1 : Gain  Gain=1/epsilon  SaturateOnIntegerOverflow=on  OutDataTypeStr=Inherit: Same as input  ParamDataTypeStr=Inherit: Same as input
  Gain2 : Gain  Gain=1/epsilon  SaturateOnIntegerOverflow=on  OutDataTypeStr=Inherit: Same as input  ParamDataTypeStr=Inherit: Same as input
  Integrator : Integrator  ExternalReset=either  InitialConditionSource=external
  Sum : Sum  Inputs=+-  SaturateOnIntegerOverflow=on  InputSameDT=on  OutDataTypeStr=Inherit: Same as first input
  Sum1 : Sum  Inputs=+-  SaturateOnIntegerOverflow=on  InputSameDT=on  OutDataTypeStr=Inherit: Same as first input
  Out : Outport
  Derivative State : Outport  Port=2
  wires:
  Integrator/1 -> Gain/1, Gain2/1, Derivative State/1
  Gain/1 -> Sum1/2
  Trigger Signal/1 -> Integrator/2
  New State/1 -> Integrator/3
  Sum1/1 -> Out/1
  Gain2/1 -> Sum/2
  Gain1/1 -> Sum1/1
  Y (t)/1 -> Sum/1, Gain1/1
  Sum/1 -> Integrator/1

== system plant2016_cybership/Data-driven controller yaw/ /look under the subsystem to see how it works ==
  note: Ficticious Reference
      | Signal of individual
      | Candidate Controller
      | R_fict (n)
  note: n - Candidate Controller Index
  Y (t) : Inport
  U (t) : Inport  Port=2
  Cost / Performance Index Generator : S-Function  FunctionName=yaw_cost_func  Parameters=w1_n, w1_d, w2_n, w2_d, C_p, C_i, C_d  SFunctionDeploymentMode=off  EnableBusSupport=off
  Demux2 : Demux  Tag=yaw_demux_2  Outputs=12
  Ficticious Reference Signal Generator : S-Function  FunctionName=yaw_fic_ref  Parameters=C_p, C_i, C_d  SFunctionDeploymentMode=off  EnableBusSupport=off
  Mux. : Mux  Inputs=2
  Mux.. : Mux  Inputs=2
  Mux2 : Mux  Tag=yaw_mux_2  Inputs=12
  To Workspace : ToWorkspace  VariableName=yaw_frs  SaveFormat=Timeseries  SampleTime=-1
  To Workspace1 : ToWorkspace  VariableName=yaw_cost  SaveFormat=Timeseries  SampleTime=-1
  Out1 : Outport
  frs : Outport  Port=2
  wires:
  U (t)/1 -> Mux../1
  Mux./1 -> Cost / Performance Index Generator/1  "(r_fict(t), u(t), y(t))"
  Mux../1 -> Ficticious Reference Signal Generator/1, Mux./1  "U & Y"
  Y (t)/1 -> Mux../2
  Ficticious Reference Signal Generator/1 -> frs/1, To Workspace/1, Demux2/1
  Mux2/1 -> Mux./2  "R_Fict ( n x 1 )"
  Cost / Performance Index Generator/1 -> To Workspace1/1, Out1/1  "Performance Index of  each candidate controller (n x 1)"
  Demux2/1 -> Mux2/1
  Demux2/2 -> Mux2/2
  Demux2/3 -> Mux2/3
  Demux2/4 -> Mux2/4
  Demux2/5 -> Mux2/5
  Demux2/6 -> Mux2/6
  Demux2/7 -> Mux2/7
  Demux2/8 -> Mux2/8
  Demux2/9 -> Mux2/9
  Demux2/10 -> Mux2/10
  Demux2/11 -> Mux2/11
  Demux2/12 -> Mux2/12

== system plant2016_cybership/Data-driven controller yaw/Adaptive  PID Controller/Approximate Derivative ==
  New State : Inport
  Trigger Signal : Inport  Port=2
  Y (t) : Inport  Port=3
  Gain : Gain  Gain=1/epsilon^2  SaturateOnIntegerOverflow=on  OutDataTypeStr=Inherit: Same as input  ParamDataTypeStr=Inherit: Same as input
  Gain1 : Gain  Gain=1/epsilon  SaturateOnIntegerOverflow=on  OutDataTypeStr=Inherit: Same as input  ParamDataTypeStr=Inherit: Same as input
  Gain2 : Gain  Gain=1/epsilon  SaturateOnIntegerOverflow=on  OutDataTypeStr=Inherit: Same as input  ParamDataTypeStr=Inherit: Same as input
  Integrator : Integrator  ExternalReset=either  InitialConditionSource=external
  Sum : Sum  Inputs=+-  SaturateOnIntegerOverflow=on  InputSameDT=on  OutDataTypeStr=Inherit: Same as first input
  Sum1 : Sum  Inputs=+-  SaturateOnIntegerOverflow=on  InputSameDT=on  OutDataTypeStr=Inherit: Same as first input
  Out : Outport
  Derivative State : Outport  Port=2
  wires:
  Sum/1 -> Integrator/1
  Y (t)/1 -> Gain1/1, Sum/1
  Gain1/1 -> Sum1/1
  Gain2/1 -> Sum/2
  Sum1/1 -> Out/1
  New State/1 -> Integrator/3
  Trigger Signal/1 -> Integrator/2
  Gain/1 -> Sum1/2
  Integrator/1 -> Derivative State/1, Gain2/1, Gain/1

== system plant2016_cybership/Environment force/Environment force1/Wind direction ==
  1st order Markov1 : Subsystem
  Band-Limited White Noise1 : simulink/Sources/Band-Limited White Noise  Cov=10  Ts=0.1  seed=[23341]
  beta_w : Outport
  wires:
  1st order Markov1/1(Out1) -> beta_w/1
  Band-Limited White Noise1/1 -> 1st order Markov1/1(In1)

== system plant2016_cybership/Environment force/Mean wind/Reference filter ==
  r(t) : Inport
  2nd order LP1 : TransferFcn  Numerator=0.4^2  Denominator=[1 2*1*0.4 0.4^2]
  r : Outport
  wires:
  r(t)/1 -> 2nd order LP1/1
  2nd order LP1/1 -> r/1

== system plant2016_cybership/Environment force/Slowly varying/1st order Markov2 ==
  In1 : Inport
  Gain : Gain  Gain=2
  Sum : Sum  Inputs=|+-
  Transfer Fcn : TransferFcn  Denominator=[50 1]
  Out1 : Outport
  wires:
  In1/1 -> Sum/1
  Sum/1 -> Transfer Fcn/1
  Transfer Fcn/1 -> Sum/2, Gain/1
  Gain/1 -> Out1/1
